simulink model "graphsage_withdelay"  (R2024b)
settings: Solver=FixedStepDiscrete  StartTime=0.0  StopTime=10  FixedStep=1  MaxStep=1  RelTol=1e-3
values from neighbouring files (symbols this model uses):
  adj = [1 1 0 0 0 0 0 0 0 0 0 0 ... (225 elements, 15x15)]    [adj_example.mat]    (also in simulink_graphsage_sample.m = padarray(adj,[maxNumNodes-sz maxNumNodes-sz],"post"))
  feats = [0.00347288744524 0.00322105130181 0.999728024006 0.00685162609443 0.0080205630511 0.0100356908515 0.00128957000561 0.00764863705263 0.002108811168 0.00117227830924 0.00645842589438 0.0083005707711 ... (15 elements, 15x1)]    [feats_example.mat]    (also in simulink_graphsage_sample.m = padarray(feats,maxNumNodes-sz,0,"post"))
  parameters = quantizeParams(parameters)    [simulink_graphsage_sample.m]
  sz = height(feats)    [simulink_graphsage_sample.m]
settings Model: Creator=ccrovell  LastModifiedBy=colin

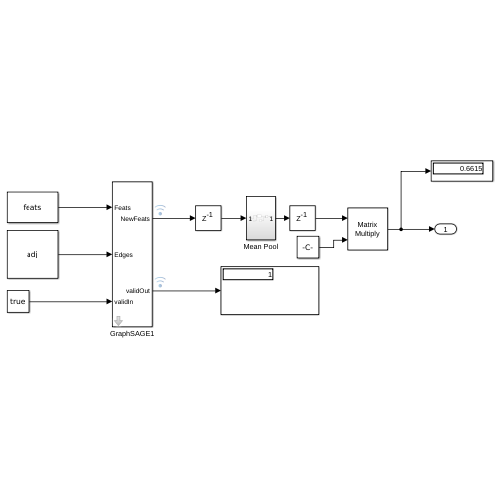
[thumbnail: Simulink's stored preview of the top-level diagram]
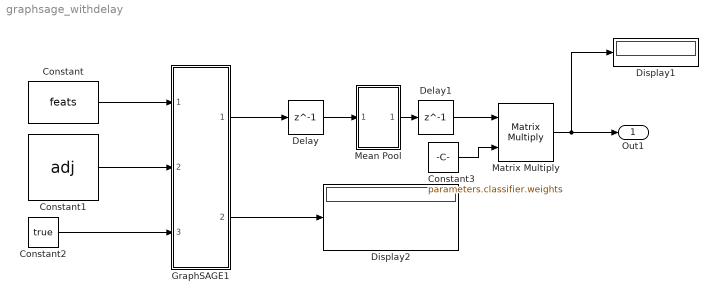
== system graphsage_withdelay ==
  Constant : Constant  Value=feats  VectorParams1D=off  OutDataTypeStr=fixdt(1,16,10)  SampleTime=-1
  Constant1 : Constant  Value=adj  OutDataTypeStr=boolean  SampleTime=-1
  Constant2 : Constant  Value=true  OutDataTypeStr=boolean  SampleTime=-1
  Constant3 : Constant  Value=parameters.classifier.weights  SampleTime=-1
  Delay : Delay  DelayLength=1
  Delay1 : Delay  DelayLength=1
  Display1 : Display
  Display2 : Display
  GraphSAGE1 : Subsystem  mask{lin_l_weight=parameters.layer1.lin_l_weight, lin_r_weight=parameters.layer1.lin_r_weight, lin_l_bias=parameters.layer1.lin_l_bias}
      mask prompts: lin_l_weight "Simulink:blkprm_prompts:ConstConstValue"; lin_r_weight "Simulink:blkprm_prompts:ConstConstValue"; lin_l_bias "Simulink:blkprm_prompts:ConstConstValue"
      mask TypeOptions lin_l_weight: lin_l_weight/Value
      mask TypeOptions lin_r_weight: lin_r_weight/Value
      mask TypeOptions lin_l_bias: lin_l_bias/Value
      mask DialogControl lin_l_weight Prompt: Constant value:
      mask DialogControl lin_r_weight Prompt: Constant value:
      mask DialogControl lin_l_bias Prompt: Constant value:
  Matrix Multiply : Product  Multiplication=Matrix(*)
  Mean Pool : Subsystem
  Out1 : Outport
  wires:
  Constant/1 -> GraphSAGE1/1(Feats)
  Constant1/1 -> GraphSAGE1/2(Edges)
  Constant2/1 -> GraphSAGE1/3(validIn)
  GraphSAGE1/2(validOut) -> Display2/1
  Constant3/1 -> Matrix Multiply/2
  GraphSAGE1/1(NewFeats) -> Delay/1
  Delay/1 -> Mean Pool/1(In1)
  Mean Pool/1(Out1) -> Delay1/1
  Delay1/1 -> Matrix Multiply/1
  Matrix Multiply/1 -> Display1/1, Out1/1

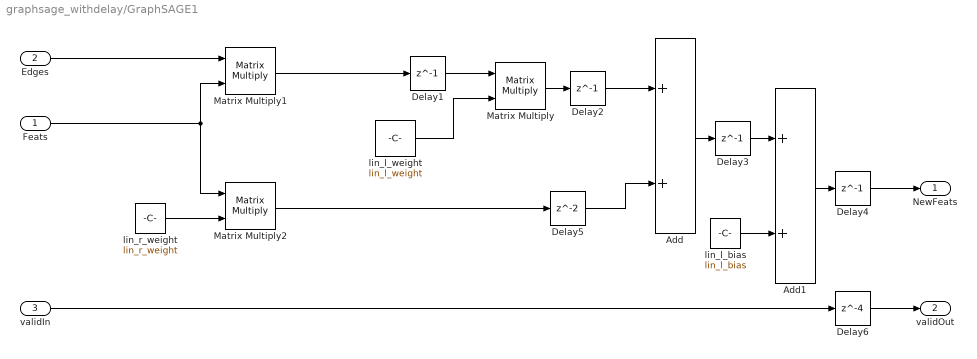
== system graphsage_withdelay/GraphSAGE1 ==
  Feats : Inport
  Edges : Inport  Port=2
  validIn : Inport  Port=3
  Add : Sum  OutDataTypeStr=Inherit: Same as first input
  Add1 : Sum  OutDataTypeStr=Inherit: Same as first input
  Delay{1..4} (4 alike) : Delay  DelayLength=1
  Delay5 : Delay
  Delay6 : Delay  DelayLength=4
  Matrix Multiply : Product  Multiplication=Matrix(*)  OutDataTypeStr=Inherit: Same as first input
  Matrix Multiply1 : Product  Multiplication=Matrix(*)  OutDataTypeStr=fixdt(1,14,10)
  Matrix Multiply2 : Product  Multiplication=Matrix(*)  OutDataTypeStr=Inherit: Same as first input
  lin_l_bias : Constant  Value=lin_l_bias  VectorParams1D=off  OutDataTypeStr=fixdt(1,16,10)  SampleTime=-1
  lin_l_weight : Constant  Value=lin_l_weight  VectorParams1D=off  OutDataTypeStr=fixdt(1,16,10)  SampleTime=-1
  lin_r_weight : Constant  Value=lin_r_weight  VectorParams1D=off  OutDataTypeStr=fixdt(1,16,10)  SampleTime=-1
  NewFeats : Outport
  validOut : Outport  Port=2
  wires:
  Add1/1 -> Delay4/1
  Add/1 -> Delay3/1
  lin_l_bias/1 -> Add1/2
  Matrix Multiply1/1 -> Delay1/1
  Matrix Multiply2/1 -> Delay5/1
  lin_r_weight/1 -> Matrix Multiply2/2
  Feats/1 -> Matrix Multiply1/2, Matrix Multiply2/1
  Edges/1 -> Matrix Multiply1/1
  Matrix Multiply/1 -> Delay2/1
  lin_l_weight/1 -> Matrix Multiply/2
  Delay1/1 -> Matrix Multiply/1
  Delay2/1 -> Add/1
  Delay3/1 -> Add1/1
  Delay4/1 -> NewFeats/1
  Delay5/1 -> Add/2
  validIn/1 -> Delay6/1
  Delay6/1 -> validOut/1

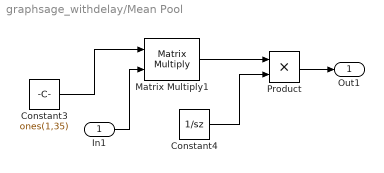
== system graphsage_withdelay/Mean Pool ==
  In1 : Inport
  Constant3 : Constant  Value=ones(1,35)  VectorParams1D=off  OutDataTypeStr=boolean  SampleTime=-1
  Constant4 : Constant  Value=1/sz  OutDataTypeStr=fixdt(1,13,10)  SampleTime=-1
  Matrix Multiply1 : Product  Multiplication=Matrix(*)
  Product : Product  OutDataTypeStr=Inherit: Same as first input
  Out1 : Outport
  wires:
  In1/1 -> Matrix Multiply1/2
  Matrix Multiply1/1 -> Product/1
  Constant4/1 -> Product/2
  Constant3/1 -> Matrix Multiply1/1
  Product/1 -> Out1/1
